simulink model "Copter_Plane_h"  (R2018b)
settings: Solver=ode1  StartTime=0.0  StopTime=20  FixedStep=dt  RelTol=1e-3
values from neighbouring files (symbols this model uses):
  center_WP = [40,100]*1e7    [Compter_Plane_inint_m_fs_form_V1028.m]    (also in Compter_Plane_inint_m_fs_form_V1029.m; Compter_Plane_inint_m_fs_form_V1030.m)
  GRAVITY_MSS = 9.80665    [Compter_Plane_inint_m_fs_form_V1028.m]    (also in Compter_Plane_inint_m_fs_form_V1029.m; Compter_Plane_inint_m_fs_form_V1030.m)
  groundspeed_vector = [0.1 0.1]    [Compter_Plane_inint_m_fs_form_V1028.m]    (also in Compter_Plane_inint_m_fs_form_V1029.m; Compter_Plane_inint_m_fs_form_V1030.m)
  gyro_x = 0    [Compter_Plane_inint_m_fs_form_V1028.m]    (also in Compter_Plane_inint_m_fs_form_V1029.m; Compter_Plane_inint_m_fs_form_V1030.m)
  gyro_y = 0    [Compter_Plane_inint_m_fs_form_V1028.m]    (also in Compter_Plane_inint_m_fs_form_V1029.m; Compter_Plane_inint_m_fs_form_V1030.m)
  gyro_z = 0    [Compter_Plane_inint_m_fs_form_V1028.m]    (also in Compter_Plane_inint_m_fs_form_V1029.m; Compter_Plane_inint_m_fs_form_V1030.m)
  HD = 180/pi    (= 57.2957795131)    [Compter_Plane_inint_m_fs_form_V1028.m]    (also in Compter_Plane_inint_m_fs_form_V1029.m; Compter_Plane_inint_m_fs_form_V1030.m)
  Kd = Ku*Luy/Ldy    (= 18.9029535865)    [Compter_Plane_inint_m_fs_form_V1028.m]    (also in Compter_Plane_inint_m_fs_form_V1029.m; Compter_Plane_inint_m_fs_form_V1030.m)
  Ku = 32    [Compter_Plane_inint_m_fs_form_V1028.m]    (also in Compter_Plane_inint_m_fs_form_V1029.m; Compter_Plane_inint_m_fs_form_V1030.m)
  Ld = hypot(Ldx,Ldy)    [Compter_Plane_inint_m_fs_form_V1028.m]    (also in Compter_Plane_inint_m_fs_form_V1029.m; Compter_Plane_inint_m_fs_form_V1030.m)
  Ldx = 205/1000    (= 0.205)    [Compter_Plane_inint_m_fs_form_V1028.m]    (also in Compter_Plane_inint_m_fs_form_V1029.m; Compter_Plane_inint_m_fs_form_V1030.m)
  Ldy = 355.5/1000    (= 0.3555)    [Compter_Plane_inint_m_fs_form_V1028.m]    (also in Compter_Plane_inint_m_fs_form_V1029.m; Compter_Plane_inint_m_fs_form_V1030.m)
  Lu = hypot(Lux,Luy)    [Compter_Plane_inint_m_fs_form_V1028.m]    (also in Compter_Plane_inint_m_fs_form_V1029.m; Compter_Plane_inint_m_fs_form_V1030.m)
  Lux = 310/1000    (= 0.31)    [Compter_Plane_inint_m_fs_form_V1028.m]    (also in Compter_Plane_inint_m_fs_form_V1029.m; Compter_Plane_inint_m_fs_form_V1030.m)
  Luy = 210/1000    (= 0.21)    [Compter_Plane_inint_m_fs_form_V1028.m]    (also in Compter_Plane_inint_m_fs_form_V1029.m; Compter_Plane_inint_m_fs_form_V1030.m)
  p_angle_pitch = 3    [Compter_Plane_inint_m_fs_form_V1028.m]    (also in Compter_Plane_inint_m_fs_form_V1029.m; Compter_Plane_inint_m_fs_form_V1030.m)
  p_angle_yaw = 3    [Compter_Plane_inint_m_fs_form_V1028.m]    (also in Compter_Plane_inint_m_fs_form_V1029.m; Compter_Plane_inint_m_fs_form_V1030.m)
  pitch = 0    [Compter_Plane_inint_m_fs_form_V1028.m]    (also in Compter_Plane_inint_m_fs_form_V1029.m; Compter_Plane_inint_m_fs_form_V1030.m)
  pwm_max = 2000    [Compter_Plane_inint_m_fs_form_V1028.m]    (also in Compter_Plane_inint_m_fs_form_V1029.m; Compter_Plane_inint_m_fs_form_V1030.m)
  pwm_min = 1000    [Compter_Plane_inint_m_fs_form_V1028.m]    (also in Compter_Plane_inint_m_fs_form_V1029.m; Compter_Plane_inint_m_fs_form_V1030.m)
  Qd = 10    [Compter_Plane_inint_m_fs_form_V1028.m]    (also in Compter_Plane_inint_m_fs_form_V1029.m; Compter_Plane_inint_m_fs_form_V1030.m)
  Qu = asind(Kd*sind(Qd)*Ld/(Ku*Lu))    [Compter_Plane_inint_m_fs_form_V1028.m]    (also in Compter_Plane_inint_m_fs_form_V1029.m; Compter_Plane_inint_m_fs_form_V1030.m)
  roll = 0    [Compter_Plane_inint_m_fs_form_V1028.m]    (also in Compter_Plane_inint_m_fs_form_V1029.m; Compter_Plane_inint_m_fs_form_V1030.m)
  throttle_hover = 0.6    [Compter_Plane_inint_m_fs_form_V1028.m]    (also in Compter_Plane_inint_m_fs_form_V1029.m; Compter_Plane_inint_m_fs_form_V1030.m)
  yaw = 0    [Compter_Plane_inint_m_fs_form_V1028.m]    (also in Compter_Plane_inint_m_fs_form_V1029.m; Compter_Plane_inint_m_fs_form_V1030.m)
undefined symbols (not defined in the file or in its folder): m
libraries: shared6dof x1, aerolibasang x1
(part 2 of 2)

== matlab function Copter_Plane_h/input_euler_angle_roll_pitch_euler_rate_yaw ==
  data: recalc_leash_z data_store_memory; leash_up_z data_store_memory; POSCONTROL_SPEED_UP data_store_memory; POSCONTROL_ACCEL_Z data_store_memory; POSCONTROL_POS_Z_P data_store_memory; leash_down_z data_store_memory; POSCONTROL_SPEED_DOWN data_store_memory; POSCONTROL_ACCELERATION_MIN data_store_memory; POSCONTROL_LEASH_LENGTH_MIN data_store_memory; limit_pos_up data_store_memory; limit_pos_down data_store_memory; pos_error data_store_memory; pos_target data_store_memory; curr_alt data_store_memory; vel_target data_store_memory; dt data_store_memory; limit_vel_up data_store_memory; limit_vel_down data_store_memory; use_desvel_ff_z data_store_memory; reset_rate_to_accel_z data_store_memory; vel_desired data_store_memory; accel_desired data_store_memory; POSCONTROL_VEL_ERROR_CUTOFF_FREQ data_store_memory; vel_last data_store_memory; freeze_ff_z data_store_memory; vel_error data_store_memory; vel_error_input data_store_memory; curr_vel data_store_memory; accel_target data_store_memory; POSCONTROL_VEL_Z_P data_store_memory; reset_accel_to_throttle data_store_memory; accel_error data_store_memory; z_accel_meas data_store_memory; pid_accel_z_reset_filter data_store_memory; POSCONTROL_ACC_Z_FILT_HZ data_store_memory; pid_accel_z_input data_store_memory; pid_accel_z_derivative data_store_memory; POSCONTROL_ACC_Z_P data_store_memory; pid_accel_z_integrator data_store_memory; POSCONTROL_ACC_Z_IMAX data_store_memory; throttle_hover data_store_memory; throttle_lower data_store_memory; throttle_upper data_store_memory; POSCONTROL_ACC_Z_D data_store_memory; throttle_input data_store_memory; POSCONTROL_ACC_Z_I data_store_memory; throttle_thrust_max data_store_memory; althold_lean_angle_max data_store_memory; angle_limit_tc data_store_memory; angle_boost_enabled data_store_memory; pitch data_store_memory; roll data_store_memory; angle_boost data_store_memory; throttle_rpy_mix data_store_memory; throttle_avg_max data_store_memory; AC_ATTITUDE_CONTROL_ANGLE_LIMIT_THROTTLE_MAX data_store_memory; POSCONTROL_POS_XY_P data_store_memory; curr_pos data_store_memory; leash data_store_memory; POSCONTROL_ACCEL_XY data_store_memory; POSCONTROL_VEL_XY_FILT_HZ data_store_memory; POSCONTROL_VEL_XY_FILT_D_HZ data_store_memory; pid_vel_xy_reset_filter data_store_memory; pid_vel_xy_input data_store_memory; pid_vel_xy_derivative data_store_memory; pid_vel_xy_integrator data_store_memory; POSCONTROL_VEL_XY_P data_store_memory; limit_accel_xy data_store_memory; motors_limit_throttle_upper data_store_memory; POSCONTROL_VEL_XY_I data_store_memory; POSCONTROL_VEL_XY_IMAX data_store_memory; POSCONTROL_VEL_XY_D data_store_memory; reset_accel_to_lean_xy data_store_memory; POSCONTROL_ACCEL_FILTER_HZ data_store_memory; accel_xy_input data_store_memory; accel_xy_angle_max data_store_memory; roll_target data_store_memory; pitch_target data_store_memory; GRAVITY_MSS data_store_memory; POSCONTROL_ACCEL_XY_MAX data_store_memory; yaw data_store_memory; recalc_leash_xy data_store_memory; POSCONTROL_SPEED data_store_memory; reset_desired_vel_to_pos data_store_memory; POSCONTROL_OVERSPEED_GAIN_Z data_store_memory; POSCONTROL_JERK_RATIO data_store_memory; accel_last_z_cms data_store_memory; is_active_z data_store_memory; POSCONTROL_STOPPING_DIST_DOWN_MAX data_store_memory; POSCONTROL_STOPPING_DIST_UP_MAX data_store_memory; is_active_xy data_store_memory; rot_body_to_ned data_store_memory; attitude_target_quat data_store_memory; attitude_target_ang_vel data_store_memory; thrust_error_angle data_store_memory; rate_target_ang_vel data_store_memory; gyro_z data_store_memory; ang_vel_roll_max data_store_memory; ang_vel_pitch_max data_store_memory; ang_vel_yaw_max data_store_memory; AC_ATTITUDE_THRUST_ERROR_ANGLE data_store_memory; rate_bf_ff_enabled data_store_memory; attitude_ang_error data_store_memory; p_angle_yaw data_store_memory; AC_ATTITUDE_ACCEL_Y_CONTROLLER_MAX_RADSS data_store_memory; use_sqrt_controller data_store_memory; p_angle_roll data_store_memory; AC_ATTITUDE_ACCEL_RP_CONTROLLER_MIN_RADSS data_store_memory; AC_ATTITUDE_ACCEL_RP_CONTROLLER_MAX_RADSS data_store_memory; p_angle_pitch data_store_memory; accel_pitch_max data_store_memory; accel_yaw_max data_store_memory; accel_roll_max data_store_memory; AC_ATTITUDE_ACCEL_Y_CONTROLLER_MIN_RADSS data_store_memory; attitude_target_euler_angle data_store_memory; input_tc data_store_memory; attitude_target_euler_rate data_store_memory; slew_yaw data_store_memory; rate_pitch_pid_reset_filter data_store_memory; rate_pitch_pid_input data_store_memory; rate_pitch_pid_derivative data_store_memory; rate_pitch_pid_integrator data_store_memory; motors_limit_roll_pitch data_store_memory; ATC_RAT_PIT_D data_store_memory; ATC_RAT_PIT_FF data_store_memory; ATC_RAT_PIT_FILT data_store_memory; ATC_RAT_PIT_I data_store_memory; ATC_RAT_PIT_IMAX data_store_memory; ATC_RAT_PIT_P data_store_memory; ATC_RAT_RLL_D data_store_memory; ATC_RAT_RLL_FF data_store_memory; ATC_RAT_RLL_FILT data_store_memory; ATC_RAT_RLL_I data_store_memory; ATC_RAT_RLL_IMAX data_store_memory; ATC_RAT_RLL_P data_store_memory; rate_roll_pid_reset_filter data_store_memory; rate_roll_pid_input data_store_memory; rate_roll_pid_derivative data_store_memory; rate_roll_pid_integrator data_store_memory; ATC_RAT_YAW_D data_store_memory; ATC_RAT_YAW_FF data_store_memory; ATC_RAT_YAW_FILT data_store_memory; ATC_RAT_YAW_I data_store_memory; ATC_RAT_YAW_IMAX data_store_memory; ATC_RAT_YAW_P data_store_memory; rate_yaw_pid_reset_filter data_store_memory; rate_yaw_pid_input data_store_memory; rate_yaw_pid_derivative data_store_memory; rate_yaw_pid_integrator data_store_memory; motors_limit_yaw data_store_memory; gyro_x data_store_memory; gyro_y data_store_memory; inint data_store_memory; AP_MOTORS_MATRIX_YAW_FACTOR_CCW data_store_memory; AP_MOTORS_MATRIX_YAW_FACTOR_CW data_store_memory; pitch_factor data_store_memory; roll_factor data_store_memory; yaw_factor data_store_memory; throttle_in data_store_memory; throttle_cutoff_frequency data_store_memory; POSCONTROL_THROTTLE_CUTOFF_FREQ data_store_memory; throttle_filter data_store_memory; armed data_store_memory; roll_in data_store_memory; pitch_in data_store_memory; yaw_in data_store_memory; thrust_boost_ratio data_store_memory; thrust_rpyt_out data_store_memory; limit_roll_pitch data_store_memory; yaw_headroom data_store_memory; thrust_boost data_store_memory; limit_yaw data_store_memory; current_tilt data_store_memory; air_density_ratio data_store_memory; pwm_max data_store_memory; pwm_min data_store_memory; thrust_slew_time data_store_memory; pwm_out data_store_memory; attitude_error_vector data_store_memory; Kx data_store_memory; target_yaw_rate data_store_memory; accel_x data_store_memory; accel_y data_store_memory; accel_z data_store_memory; climb_rate_cms data_store_memory; mode data_store_memory
function input_euler_angle_roll_pitch_euler_rate_yaw


global roll_target
global pitch_target
global target_yaw_rate
global POSCONTROL_THROTTLE_CUTOFF_FREQ
global throttle_in
global mode

global inint
    if(inint)
    setup_motors() ;
    inint=0;
    end
updata_cl();
if(mode==1)%%mode=1 alt on
 update_vel_controller_xyz()
else
set_throttle_out(throttle_in, 1, POSCONTROL_THROTTLE_CUTOFF_FREQ);
end
input_euler_angle_roll_pitch_euler_rate_yaw(  roll_target,   pitch_target,   target_yaw_rate)
rate_controller_run()


% roll_in=rate_target_to_motor_roll(  gyro_x,  0);
% pitch_in=rate_target_to_motor_pitch( gyro_y,  0);
% yaw_in=rate_target_to_motor_yaw(  gyro_z,   5);

AP_MotorsMulticopter_output()
end

== matlab function Copter_Plane_h/MATLAB Function1 ==
  data: q input; euler_angle output
function euler_angle= to_euler(q)

euler_angle= to_euler(q);

== matlab function Copter_Plane_h/MATLAB Function2 ==
  data: q input; euler_angle output
function euler_angle= to_euler(q)

euler_angle= to_euler(q);

== matlab function Copter_Plane_h/curr_vel_limt ==
  data: Ve input; Vo output; Xe input
function Vo = curr_vel_limt(Ve,Xe)

if((Xe(3)==0)&&(Ve(3)>0))
    Vo=[Ve(1) Ve(2)  0]';
else
    Vo=Ve;    
end

== matlab function Copter_Plane_h/MATLAB Function3 ==
  data: center_WP input; current_loc output; ofs_north input; ofs_east input; LOCATION_SCALING_FACTOR_INV data_store_memory; HD data_store_memory
function current_loc=Location_offset( center_WP,ofs_north,  ofs_east)

current_loc=Location_offset( center_WP,ofs_north,  ofs_east);

== matlab function Copter_Plane_h/get_servo_out ==
  data: wy data_store_memory; gains_I_pitch data_store_memory; gains_tau_pitch data_store_memory; gains_P_pitch data_store_memory; gains_D_pitch data_store_memory; gains_imax_pitch data_store_memory; gains_FF_pitch data_store_memory; airspeed_min data_store_memory; last_out_pitch data_store_memory; pid_info_I_pitch data_store_memory; pid_info_P_pitch data_store_memory; pid_info_FF_pitch data_store_memory; pid_info_D_pitch data_store_memory; pid_info_desired_pitch data_store_memory; pid_info_actual_pitch data_store_memory; roll data_store_memory; pitch data_store_memory; roll_limit_cd data_store_memory; aspeed data_store_memory; max_rate_neg data_store_memory; gains_rmax_pitch data_store_memory; GRAVITY_MSS data_store_memory; roll_ff_pitch data_store_memory; HD data_store_memory; gains_D_roll data_store_memory; gains_FF_roll data_store_memory; gains_I_roll data_store_memory; gains_imax_roll data_store_memory; gains_P_roll data_store_memory; gains_rmax_roll data_store_memory; gains_tau_roll data_store_memory; last_out_roll data_store_memory; pid_info_actual_roll data_store_memory; pid_info_D_roll data_store_memory; pid_info_desired_roll data_store_memory; pid_info_FF_roll data_store_memory; pid_info_I_roll data_store_memory; pid_info_P_roll data_store_memory; wx data_store_memory; accel_y data_store_memory; imax_yaw data_store_memory; integrator_yaw data_store_memory; K_A_yaw data_store_memory; K_D_last_yaw data_store_memory; K_D_yaw data_store_memory; K_FF_yaw data_store_memory; K_I_yaw data_store_memory; last_out_yaw data_store_memory; last_rate_hp_in_yaw data_store_memory; last_rate_hp_out_yaw data_store_memory; pid_info_D_yaw data_store_memory; pid_info_I_yaw data_store_memory; wz data_store_memory; throttle_dem data_store_memory; pitch_dem data_store_memory; pitch_limit_min_cd data_store_memory; pitch_limit_max_cd data_store_memory; nav_pitch_cd data_store_memory; nav_roll_cd data_store_memory; inverted_flight data_store_memory; k_rudder data_store_memory; k_aileron data_store_memory; k_throttle data_store_memory; k_elevator data_store_memory; kff_throttle_to_pitch data_store_memory; highest_airspeed data_store_memory; scaling_speed data_store_memory; airspeed_max data_store_memory; latAccDem data_store_memory; smoothed_airspeed data_store_memory; aerodynamic_load_factor data_store_memory; kff_rudder_mix data_store_memory; hgt_dem_cm input; EAS_dem_cm input; TASmax data_store_memory; SKE_dem data_store_memory; TASmin data_store_memory; SPE_dem data_store_memory; SPE_est data_store_memory; SKE_est data_store_memory; STE_error data_store_memory; SPEdot_dem data_store_memory; SKEdot_dem data_store_memory; STEdot_min data_store_memory; STEdot_max data_store_memory; SPEdot data_store_memory; SKEdot data_store_memory; STEdotErrLast data_store_memory; timeConstant data_store_memory; throttle_cruise data_store_memory; rot_body_to_ned data_store_memory; rollComp data_store_memory; THRmaxf data_store_memory; THRminf data_store_memory; thrDamp data_store_memory; throttle_slewrate data_store_memory; last_throttle_dem data_store_memory; integGain data_store_memory; integTHR_state data_store_memory; maxClimbRate data_store_memory; minSinkRate data_store_memory; EAS_dem data_store_memory; hgt_dem data_store_memory; throttle_max data_store_memory; throttle_min data_store_memory; pitch_max data_store_memory; PITCHmaxf data_store_memory; pitch_min data_store_memory; PITCHminf data_store_memory; pitch_max_limit data_store_memory; TAS_dem data_store_memory; EAS2TAS data_store_memory; EAS data_store_memory; TAS_state data_store_memory; integDTAS_state data_store_memory; spdCompFiltOmega data_store_memory; vel_dot data_store_memory; TAS_dem_adj data_store_memory; TAS_rate_dem data_store_memory; hgt_dem_in_old data_store_memory; maxSinkRate data_store_memory; hgt_dem_prev data_store_memory; hgt_dem_adj_last data_store_memory; hgt_dem_adj data_store_memory; hgt_rate_dem data_store_memory; height data_store_memory; climb_rate data_store_memory; spdWeight data_store_memory; ptchDamp data_store_memory; pitch_dem_unc data_store_memory; integSEB_state data_store_memory; vertAccLim data_store_memory; last_pitch_dem data_store_memory; center_WP input; radius input; loiter_direction input; prev_WP input; next_WP input; dist_min input; L1_damping data_store_memory; L1_period data_store_memory; current_loc data_store_memory; groundspeed_vector data_store_memory; target_bearing_cd data_store_memory; L1_dist data_store_memory; crosstrack_error data_store_memory; nav_bearing data_store_memory; L1_xtrack_i_gain data_store_memory; L1_xtrack_i_gain_prev data_store_memory; L1_xtrack_i data_store_memory; last_Nu data_store_memory; WPcircle data_store_memory; data_is_stale data_store_memory; bearing_error data_store_memory; LOCATION_SCALING_FACTOR data_store_memory; yaw data_store_memory; reverse data_store_memory; loiter_bank_limit data_store_memory; dt data_store_memory; roll_limit_cd_inint data_store_memory; accel_x data_store_memory; accel_z data_store_memory; Vz data_store_memory; vdot_filter data_store_memory; pwm_min data_store_memory; pwm_max data_store_memory; pwm_out data_store_memory; LOCATION_SCALING_FACTOR_INV data_store_memory
function get_servo_out(   hgt_dem_cm, EAS_dem_cm, center_WP,   radius,   loiter_direction,prev_WP,  next_WP,  dist_min)
global aerodynamic_load_factor
global current_loc
updata_cl();
update_50hz();
update_pitch_throttle(  hgt_dem_cm,EAS_dem_cm,aerodynamic_load_factor)
update_loiter( center_WP,   radius,   loiter_direction)
% update_waypoint( prev_WP,  next_WP,  dist_min)
% update_loiter( center_WP,   radius,   loiter_direction)
% update_waypoint( prev_WP,  next_WP,  dist_min)
% update_pitch_throttle(  hgt_dem_cm,EAS_dem_cm,load_factor)
calc_nav_pitch();
calc_nav_roll()
calc_throttle()
stabilize()
output_to_motors_plane();

== matlab function Copter_Plane_h/pland_F_M ==
  data: F output; k_rudder input; k_aileron input; k_throttle input; k_elevator input; wx input; wy input; wz input; alpha input; beta input; V input; alt input; M output; mode input; pwm_out input; Ku parameter; Kd parameter; Lux parameter; Luy parameter; Ldx parameter; Ldy parameter; Lu parameter; Ld parameter; pwm_min parameter; pwm_max parameter; Qu parameter; Qd parameter
function [F,M]   = pland_F_M(k_rudder,k_aileron,k_throttle,k_elevator,wx,wy,wz,alpha,beta,V,alt,mode,pwm_out, Ku, Kd, Lux, Luy, Ldx, Ldy, Lu, Ld, pwm_min, pwm_max, Qu, Qd)
    
%推力模型，Thr=throttle_dem*Tmax，throttle_dem=24N。
%阻力模型，Cx_Sref=Cx_Sref_alpha*alpha,Cx_Sref_alpha=0.007;
%升力模型  Cy_Sref=Cy_Sref_alpha*(alpha0+alpha),Cy_Sref_alpha=0.022,alpha0=5;
%%%%%%%%%%%%%%%%%%%%%%%%%%%%%%%%%%%%%%%%%%%%%%%%%%%%%%%%%%%%%%%%%%%%%%%
Tmax=36;
HD=180/pi;
Cx_Sref_alpha=-0.0554;%8/144.5
Cz_Sref_alpha=-0.1075*0.86;
Cy_Sref_beta=-0.1075*0.86*0.1;
alpha0=2/HD;
Cx_Sref=Cx_Sref_alpha;
Cy_Sref=Cy_Sref_beta*(beta)*HD;
Cz_Sref=Cz_Sref_alpha*(alpha+alpha0)*HD;

Sbw=[cos(alpha)*cos(beta)   -cos(alpha)*sin(beta)   -sin(alpha)
    sin(beta)               cos(beta)               0
    sin(alpha)*cos(beta)    -sin(alpha)*sin(beta)   cos(alpha)];
[~,~,rho,~] = atom_mode(alt+2000);
q=0.5*rho*V*V;
D=q*Cx_Sref;%+k_throttle*Tmax;
C=q*Cy_Sref;
L=q*Cz_Sref;
Fw=[D; C; L];

Fb=Sbw*Fw;
F_Plane=Fb+[k_throttle*Tmax;0;0];
%%%%%%%%%%%%%%%%%%%%%%%%%%%%%%%%%%%%%%%%%%%%%%%%%
dl=0.1;
Mby=Fb(3)*dl;
Mbz=-Fb(2)*dl;
%%%%%%%%%%%%%%%%%%%%%%%%%
dmxa=3.2078;    %(2*pi*5)^2*Jx/HD
dmx_wx=0.1;
%%%%%%%%%%%%%%%%%%%%%%%%%%%
dmya=q*Cz_Sref_alpha*dl;  %(2*pi*1.5)^2*Jy/HD
dmye=-dmya/2;
dmy_wy=0.2;
%%%%%%%%%%%%%%%%%%%%%%%%%
dmzb=-q*Cy_Sref_beta*dl;    %(2*pi*5)^2*Jx/HD
dmzr=dmzb*0.3;
dmz_wz=0.2;
%%%%%%%%%%%%%%%%%%%%%%%%
Mx=dmxa*k_aileron/100          -dmx_wx*wx;
My=dmye*(k_elevator+680)/100  +Mby   -dmy_wy*wy;
Mz=dmzr*k_rudder/100    +Mbz   -dmz_wz*wz;
M_Plane=[Mx; My ;Mz];
%%%%%%%%%%%%%%%%%%%%%%%%%%%%%%%%%%%%%%%%%%%%%%%%%%%%%%%%%%%%%%%%%%%
%%%%%%%%%%%%%%%%%%%%%%%%%%%%%%%%%%%%%%%%%%%%%%%%%%%%%%%%%%%%%%%%%%%%%
F1=(pwm_out(1)-pwm_min)/(pwm_max-pwm_min)*Ku;
F2=(pwm_out(2)-pwm_min)/(pwm_max-pwm_min)*Kd;
F3=(pwm_out(3)-pwm_min)/(pwm_max-pwm_min)*Ku;
F4=(pwm_out(4)-pwm_min)/(pwm_max-pwm_min)*Kd;

F_copter=-[0; 0 ;F1+F2+F3+F4];
Mx=(-F1+F3)*Lux+(F2-F4)*Ldx;
My=(F1+F3)*Luy+(-F2-F4)*Ldy;
Mz=(-F1+F3)*Lu*sind(Qu)+(-F2+F4)*Ld*sind(Qd);%0.1736=sind(10)  0.1071= Ld*900*sind(10)/(Lu*1600)
M_copter=[Mx; My; Mz];
%%%%%%%%%%%%%%%%%%%%%%%%%%%%%%%%%%%%%%%%%%%%%%%%%%%%%%%
%% 0 :copter Stabilize,1:copter althold ,2:copter poshold,3:Plane Stabilize 4:Plane TECS; 5：Plane L1
F=[0 ;0 ;0];
M=[0 ;0 ;0];
if(mode==0||mode==1||mode==2)
    F=F_copter;
    M=M_copter;
else
    F=F_Plane;
    M=M_Plane;
end
%%%%%%%%%%%%%%%%%%%%%%%%%%%%%%%%%%%%%%%%%%%%%%%%%%%%%%%%%%%%

end
